simulink model "switch_case_test"  (Simulink 8.4)
settings: Solver=VariableStepDiscrete  StartTime=0.0  StopTime=1  MaxStep=1  RelTol=1e-3
settings Model: Creator=arnaud  LastModifiedBy=arnaud
settings DataIOCC: SaveFormat=Structure  SignalLoggingSaveFormat=Dataset
settings OptimizationCC: ExpressionDepthLimit=128
settings DebuggingCC: UnderspecifiedInitializationDetection=Simplified  MergeDetectMultiDrivingBlocksExec=error  FcnCallInpInsideContextMsg=EnableAllAsError  StateNameClashWarn=none
settings GRTTargetCC: CombineOutputUpdateFcns=on  GRTInterface=off

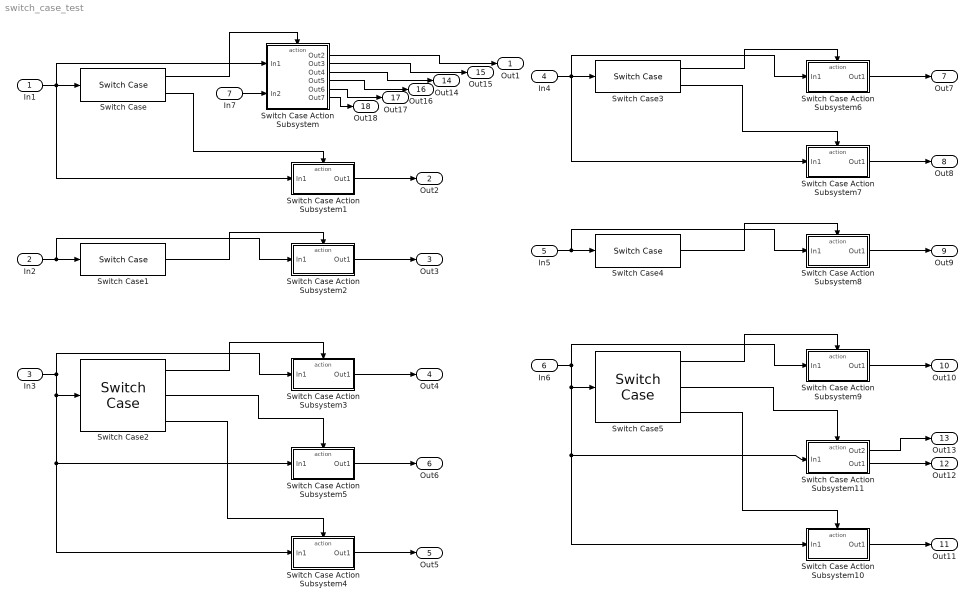
== system switch_case_test ==
  In1 : Inport
  In2 : Inport  Port=2
  In3 : Inport  Port=3
  In4 : Inport  Port=4  OutDataTypeStr=int32
  In5 : Inport  Port=5  OutDataTypeStr=int32
  In6 : Inport  Port=6  OutDataTypeStr=int32
  In7 : Inport  Port=7  OutDataTypeStr=boolean
  Switch Case : SwitchCase
  Switch Case Action Subsystem : Subsystem  TreatAsAtomicUnit=on
  Switch Case Action Subsystem1 : Subsystem  TreatAsAtomicUnit=on
  Switch Case Action Subsystem10 : Subsystem  TreatAsAtomicUnit=on
  Switch Case Action Subsystem11 : Subsystem  TreatAsAtomicUnit=on
  Switch Case Action Subsystem2 : Subsystem  TreatAsAtomicUnit=on
  Switch Case Action Subsystem3 : Subsystem  TreatAsAtomicUnit=on
  Switch Case Action Subsystem4 : Subsystem  TreatAsAtomicUnit=on
  Switch Case Action Subsystem5 : Subsystem  TreatAsAtomicUnit=on
  Switch Case Action Subsystem6 : Subsystem  TreatAsAtomicUnit=on
  Switch Case Action Subsystem7 : Subsystem  TreatAsAtomicUnit=on
  Switch Case Action Subsystem8 : Subsystem  TreatAsAtomicUnit=on
  Switch Case Action Subsystem9 : Subsystem  TreatAsAtomicUnit=on
  Switch Case1 : SwitchCase  ShowDefaultCase=off
  Switch Case2 : SwitchCase  CaseConditions={1,[2,5]}
  Switch Case3 : SwitchCase
  Switch Case4 : SwitchCase  ShowDefaultCase=off
  Switch Case5 : SwitchCase  CaseConditions={1,[2,5]}
  Out1 : Outport
  Out2 : Outport  Port=2
  Out3 : Outport  Port=3
  Out4 : Outport  Port=4
  Out5 : Outport  Port=5
  Out6 : Outport  Port=6
  Out7 : Outport  Port=7
  Out8 : Outport  Port=8
  Out9 : Outport  Port=9
  Out10 : Outport  Port=10
  Out11 : Outport  Port=11
  Out12 : Outport  Port=12
  Out13 : Outport  Port=13
  Out14 : Outport  Port=14
  Out15 : Outport  Port=15
  Out16 : Outport  Port=16
  Out17 : Outport  Port=17
  Out18 : Outport  Port=18
  wires:
  In1/1 -> Switch Case Action Subsystem/1(In1), Switch Case Action Subsystem1/1(In1), Switch Case/1
  Switch Case/1 -> Switch Case Action Subsystem/Action
  Switch Case/2 -> Switch Case Action Subsystem1/Action
  Switch Case Action Subsystem/1(Out2) -> Out1/1
  Switch Case Action Subsystem1/1(Out1) -> Out2/1
  In2/1 -> Switch Case Action Subsystem2/1(In1), Switch Case1/1
  Switch Case1/1 -> Switch Case Action Subsystem2/Action
  Switch Case Action Subsystem2/1(Out1) -> Out3/1
  In3/1 -> Switch Case Action Subsystem5/1(In1), Switch Case Action Subsystem4/1(In1), Switch Case2/1, Switch Case Action Subsystem3/1(In1)
  Switch Case2/1 -> Switch Case Action Subsystem3/Action
  Switch Case2/3 -> Switch Case Action Subsystem4/Action
  Switch Case Action Subsystem3/1(Out1) -> Out4/1
  Switch Case Action Subsystem4/1(Out1) -> Out5/1
  Switch Case Action Subsystem5/1(Out1) -> Out6/1
  Switch Case2/2 -> Switch Case Action Subsystem5/Action
  In4/1 -> Switch Case Action Subsystem7/1(In1), Switch Case Action Subsystem6/1(In1), Switch Case3/1
  Switch Case3/1 -> Switch Case Action Subsystem6/Action
  Switch Case3/2 -> Switch Case Action Subsystem7/Action
  Switch Case Action Subsystem6/1(Out1) -> Out7/1
  Switch Case Action Subsystem7/1(Out1) -> Out8/1
  In5/1 -> Switch Case Action Subsystem8/1(In1), Switch Case4/1
  Switch Case4/1 -> Switch Case Action Subsystem8/Action
  Switch Case Action Subsystem8/1(Out1) -> Out9/1
  In6/1 -> Switch Case Action Subsystem11/1(In1), Switch Case Action Subsystem10/1(In1), Switch Case5/1, Switch Case Action Subsystem9/1(In1)
  Switch Case5/1 -> Switch Case Action Subsystem9/Action
  Switch Case5/3 -> Switch Case Action Subsystem10/Action
  Switch Case Action Subsystem9/1(Out1) -> Out10/1
  Switch Case Action Subsystem10/1(Out1) -> Out11/1
  Switch Case Action Subsystem11/2(Out1) -> Out12/1
  Switch Case5/2 -> Switch Case Action Subsystem11/Action
  Switch Case Action Subsystem11/1(Out2) -> Out13/1
  In7/1 -> Switch Case Action Subsystem/2(In2)
  Switch Case Action Subsystem/2(Out3) -> Out15/1
  Switch Case Action Subsystem/3(Out4) -> Out14/1
  Switch Case Action Subsystem/4(Out5) -> Out16/1
  Switch Case Action Subsystem/5(Out6) -> Out17/1
  Switch Case Action Subsystem/6(Out7) -> Out18/1

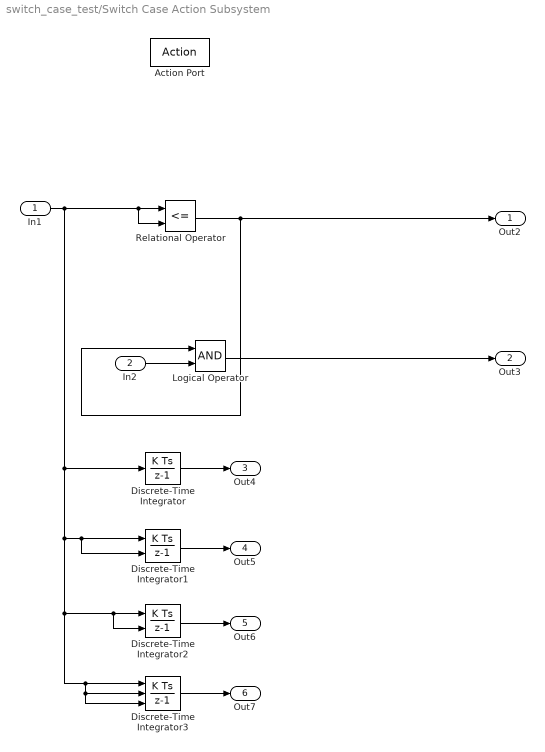
== system switch_case_test/Switch Case Action Subsystem ==
  In1 : Inport
  In2 : Inport  Port=2
  Action Port : ActionPort  InitializeStates=reset  ActionType=case
  Discrete-Time Integrator : DiscreteIntegrator  InitialConditionSetting=State (most efficient)
  Discrete-Time Integrator1 : DiscreteIntegrator  ExternalReset=falling  InitialConditionSetting=State (most efficient)
  Discrete-Time Integrator2 : DiscreteIntegrator  InitialConditionSource=external  InitialConditionSetting=State (most efficient)
  Discrete-Time Integrator3 : DiscreteIntegrator  ExternalReset=level  InitialConditionSource=external  InitialConditionSetting=State (most efficient)
  Logical Operator : Logic  AllPortsSameDT=off  OutDataTypeStr=boolean
  Relational Operator : RelationalOperator  Operator=<=  OutDataTypeStr=boolean
  Out2 : Outport
  Out3 : Outport  Port=2
  Out4 : Outport  Port=3
  Out5 : Outport  Port=4
  Out6 : Outport  Port=5
  Out7 : Outport  Port=6
  wires:
  In1/1 -> Relational Operator/1, Relational Operator/2, Discrete-Time Integrator1/2, Discrete-Time Integrator1/1, Discrete-Time Integrator2/2, Discrete-Time Integrator2/1, Discrete-Time Integrator3/3, Discrete-Time Integrator3/2, Discrete-Time Integrator3/1, Discrete-Time Integrator/1
  Relational Operator/1 -> Logical Operator/1, Out2/1
  In2/1 -> Logical Operator/2
  Logical Operator/1 -> Out3/1
  Discrete-Time Integrator/1 -> Out4/1
  Discrete-Time Integrator1/1 -> Out5/1
  Discrete-Time Integrator2/1 -> Out6/1
  Discrete-Time Integrator3/1 -> Out7/1

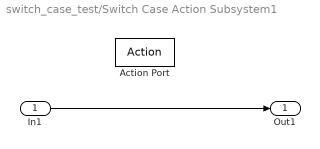
== system switch_case_test/Switch Case Action Subsystem1 ==
  In1 : Inport
  Action Port : ActionPort  ActionType=default
  Out1 : Outport
  wires:
  In1/1 -> Out1/1

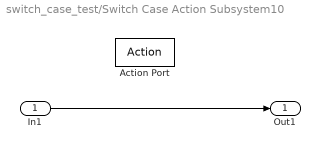
== system switch_case_test/Switch Case Action Subsystem10 ==
  In1 : Inport
  Action Port : ActionPort  ActionType=default
  Out1 : Outport
  wires:
  In1/1 -> Out1/1

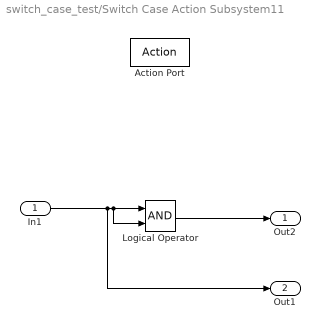
== system switch_case_test/Switch Case Action Subsystem11 ==
  In1 : Inport
  Action Port : ActionPort  ActionType=case
  Logical Operator : Logic  AllPortsSameDT=off  OutDataTypeStr=boolean
  Out2 : Outport
  Out1 : Outport  Port=2
  wires:
  In1/1 -> Logical Operator/1, Logical Operator/2, Out1/1
  Logical Operator/1 -> Out2/1

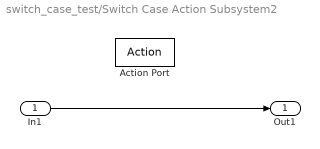
== system switch_case_test/Switch Case Action Subsystem2 ==
  In1 : Inport
  Action Port : ActionPort  ActionType=case
  Out1 : Outport
  wires:
  In1/1 -> Out1/1

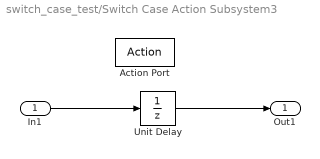
== system switch_case_test/Switch Case Action Subsystem3 ==
  In1 : Inport
  Action Port : ActionPort  InitializeStates=reset  ActionType=case
  Unit Delay : UnitDelay  SampleTime=-1
  Out1 : Outport
  wires:
  In1/1 -> Unit Delay/1
  Unit Delay/1 -> Out1/1

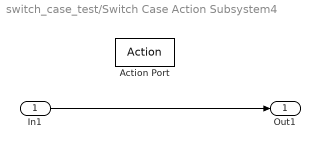
== system switch_case_test/Switch Case Action Subsystem4 ==
  In1 : Inport
  Action Port : ActionPort  ActionType=default
  Out1 : Outport
  wires:
  In1/1 -> Out1/1

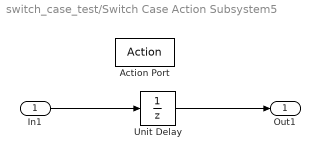
== system switch_case_test/Switch Case Action Subsystem5 ==
  In1 : Inport
  Action Port : ActionPort  ActionType=case
  Unit Delay : UnitDelay  SampleTime=-1
  Out1 : Outport
  wires:
  In1/1 -> Unit Delay/1
  Unit Delay/1 -> Out1/1

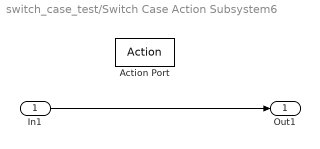
== system switch_case_test/Switch Case Action Subsystem6 ==
  In1 : Inport
  Action Port : ActionPort  ActionType=case
  Out1 : Outport
  wires:
  In1/1 -> Out1/1

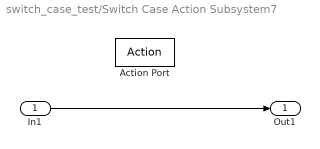
== system switch_case_test/Switch Case Action Subsystem7 ==
  In1 : Inport
  Action Port : ActionPort  ActionType=default
  Out1 : Outport
  wires:
  In1/1 -> Out1/1

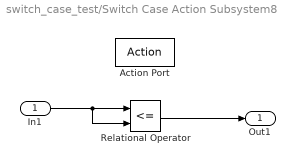
== system switch_case_test/Switch Case Action Subsystem8 ==
  In1 : Inport
  Action Port : ActionPort  ActionType=case
  Relational Operator : RelationalOperator  Operator=<=  OutDataTypeStr=boolean
  Out1 : Outport
  wires:
  In1/1 -> Relational Operator/1, Relational Operator/2
  Relational Operator/1 -> Out1/1

== system switch_case_test/Switch Case Action Subsystem9 ==
  In1 : Inport
  Action Port : ActionPort  ActionType=case
  Out1 : Outport
  wires:
  In1/1 -> Out1/1
